simulink model "simu"  (R2016b)
settings: Solver=FixedStepAuto  StartTime=0.0  StopTime=t_max  FixedStep=timestep  RelTol=1e-3
values from neighbouring files (symbols this model uses):
  Cd = 5    [script.m]
  g = 9.81    [script.m]
  L = 8e-2    (= 0.08)    [script.m]
  step_v = 0.4    [script.m]
  upstreamHeight = 0.4    [script.m]
undefined symbols (not defined in the file or in its folder): denD, numD
settings Model: Creator=mluser  LastModifiedBy=Gabriel
settings DataIOCC: ReturnWorkspaceOutputs=on
settings DebuggingCC: UnconnectedInputMsg=none  UnconnectedOutputMsg=none  UnconnectedLineMsg=none
settings ModelReferenceCC: EnableRefExpFcnMdlSchedulingChecks=off
settings SFSimCC: SimUseLocalCustomCode=on
settings RTWCC: RTWUseLocalCustomCode=on

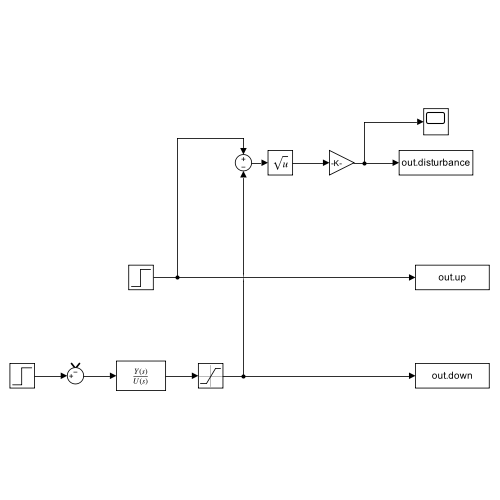
[thumbnail: Simulink's stored preview of the top-level diagram]
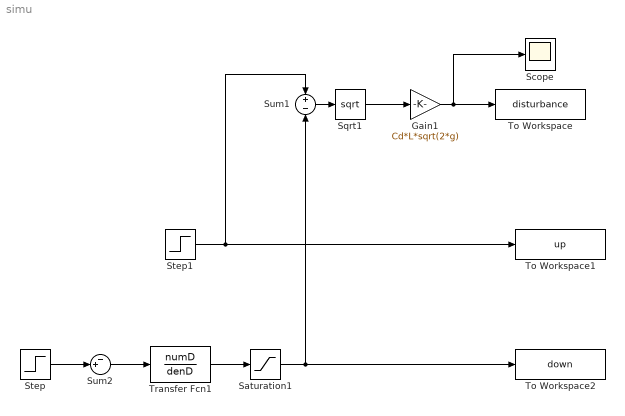
== system simu ==
  Gain1 : Gain  Gain=Cd*L*sqrt(2*g)
  Saturation1 : Saturate  UpperLimit=inf  LowerLimit=0
  Scope : Scope
  Sqrt1 : Sqrt  SaturateOnIntegerOverflow=on
  Step : Step  After=step_v  SampleTime=0
  Step1 : Step  After=upstreamHeight  SampleTime=0
  Sum1 : Sum  Inputs=+|-
  Sum2 : Sum  Inputs=-+|
  To Workspace : ToWorkspace  VariableName=disturbance  SampleTime=-1
  To Workspace1 : ToWorkspace  VariableName=up  SampleTime=-1
  To Workspace2 : ToWorkspace  VariableName=down  SampleTime=-1
  Transfer Fcn1 : TransferFcn  Numerator=numD  Denominator=denD
  wires:
  Sqrt1/1 -> Gain1/1
  Transfer Fcn1/1 -> Saturation1/1
  Sum1/1 -> Sqrt1/1
  Gain1/1 -> To Workspace/1, Scope/1
  Step1/1 -> To Workspace1/1, Sum1/1
  Saturation1/1 -> To Workspace2/1, Sum1/2
  Step/1 -> Sum2/2
  Sum2/1 -> Transfer Fcn1/1
